simulink model "ps_model"  (R2023b)
settings: Solver=ode23tb  StartTime=0.0  StopTime=simlength  FixedStep=tc  MaxStep=tc
undefined symbols (not defined in the file): Amplitude_U, Amplitude_V, Amplitude_W, CFi, end_time_LVRT, fnom, fPWM_INV, i_nom, ki_i, ki_u, kp_i, kp_u, Ld2_trafo_out, magnitude, n10, number_of_cells, omega_grid_emulator_nom, Phase_shift, Q, q1Kalman, q2Kalman, q3Kalman, R_RLload, Rd2_trafo_out, rKalman, start_time_LVRT, t_ramp, tc, time_load_step, ts_afe, ts_inv, tsample, u_nom, ugrid_factor, V_phase_normalization_factor, Vdc_base, Vdc_nom, Vemu_ref_norm, vn_eta_pu, vn_xi_pu, vp_xi_pu
libraries: fl_lib x120, nesl_utility x67, cstblocks x8, ee_lib x7, single_phase_transformer_lib x3, lithium_ion_cell_lib x1, simulink x1, threephase_inductor_lib x1
(part 1 of 4)
settings Model: SimulationMode=accelerator  Creator=dbagn  LastModifiedBy=dbagn
settings SolverCC: NumberNewtonIterations=3  ZeroCrossControl=DisableAll  AlgebraicLoopSolver=TrustRegion  SolverResetMethod=Robust
settings DataIOCC: SaveOutput=off  SignalLogging=off  DSMLogging=off  SaveTime=off  ReturnWorkspaceOutputs=off
settings OptimizationCC: ReuseModelBlockBuffer=off
settings DebuggingCC: UnconnectedInputMsg=warning  UnconnectedOutputMsg=warning  UnconnectedLineMsg=warning
settings ModelReferenceCC: EnableRefExpFcnMdlSchedulingChecks=on
settings SFSimCC: SimUserIncludeDirs=include  SimAnalyzeCustomCode=on
settings SFSimCC: SimCustomHeaderCode=|
  | #include "mavgflt.h"
  | #include "bemf_obsv.h"
  | #include "dqvector_pi.h"
  | #include "dqvector_pi_simulink.h"
  | #include "mavgflt_simulink.h"
  | #include "sv_pwm.h"
  | #include "bemf_obsv_simulink.h"
  | #include "bemf_obsv_redu.h"
  | #include "bemf_obsv_redu_simulink.h"
  | #include "bemf_obsv_load_est.h"
  | #include "bemf_obsv_load_est_simulink.h"
  | #include "bemf_obsv_load_est_redu.h"
  | #include "bemf_obsv_load_est_redu_simulink.h"
  | #include "sv_pwm_simulink.h"
  | #include "fb_state_machine.h"
  | #include "fb_state_machine_simulink.h"
settings SFSimCC: SimUserSources=|
  | dqvector_pi.c
  | dqvector_pi_simulink.c
  | mavgflt_simulink.c
  | mavgflt.c
  | bemf_obsv_simulink.c
  | bemf_obsv.c
  | bemf_obsv_redu_simulink.c
  | bemf_obsv_redu.c
  | bemf_obsv_load_est_simulink.c
  | bemf_obsv_load_est.c
  | bemf_obsv_load_est_redu_simulink.c
  | bemf_obsv_load_est_redu.c
  | sv_pwm.c
  | sv_pwm_simulink.c
  | fb_state_machine.c
  | fb_state_machine_simulink.c
settings RTWCC: DLArmComputeVersion=19.05

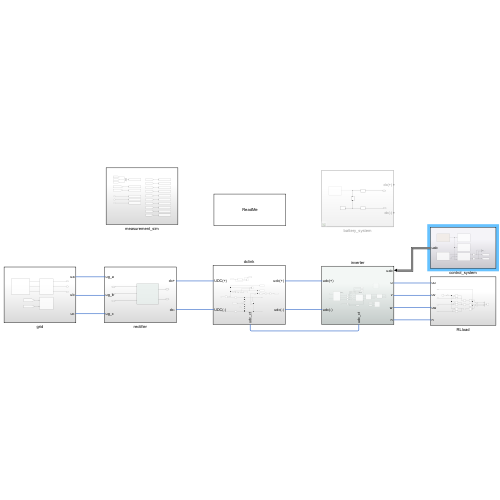
[thumbnail: Simulink's stored preview of the top-level diagram]
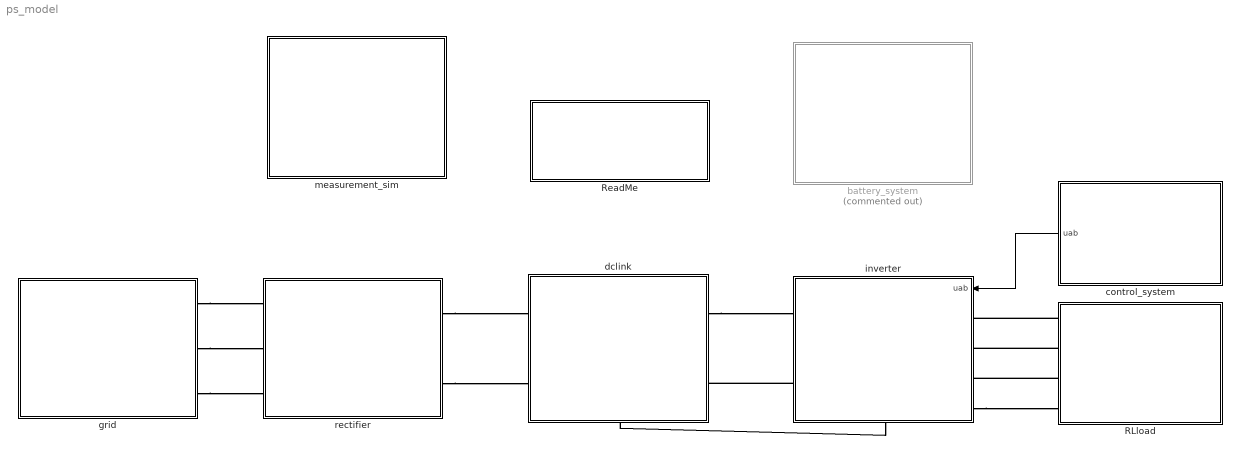
== system ps_model ==
  RLload : Subsystem
  ReadMe : Subsystem
      mask Display: disp('ReadMe')
  battery_system : Subsystem  Commented=on
  control_system : Subsystem
  dclink : Subsystem
      settings: PortSchema="{\"entries\":[{\"content\":{\"sides\":[{\"content\":{\"connectorIds\":[\"LConn1\",\"LConn2\"]},\"type\":\"ConnectorPlacement.EquallySpacedRectSide\",\"uuid\":\"065d3cf8-4b88-4bd8-afed-5c791b4c8227\"},{\"content\":{\"connectorIds\":[\"RConn1\",\"RConn2\"],\"side\":\"RIGHT\"},\"type\":\"ConnectorPlacement.EquallySpacedRectSide\",\"uuid\":\"93da4eee-d833-4749-b194-724bf2a8184c\"},{\"content\":{\"side\":\"TOP\"},\"type\":\"ConnectorPlacement.EquallySpacedRectSide\",\"uuid\":\"7e72ab0b-6fa9-40de-a645-1ec9cfd9e31f\"},{\"content\":{\"connectorIds\":[\"RConn3\"],\"side\":\"BOTTOM\"},\"type\":\"ConnectorPlacement.EquallySpacedRectSide\",\"uuid\":\"310375c4-299b-412a-a0fa-962bdc2b4f11\"}]},\"type\":\"ConnectorPlacement.EquallySpacedConnector\",\"uuid\":\"547429aa-4b93-405e-bc45-7aab171afd7d\"}],\"packageUris\":[\"http://schema.mathworks.com/mf0/Connector/R2020b\"],\"version\":\"1.0\"}"
  grid : Subsystem
  inverter : Subsystem
      settings: PortSchema="{\"entries\":[{\"content\":{\"sides\":[{\"content\":{\"connectorIds\":[\"In1\",\"LConn1\",\"LConn2\",\"LConn3\",\"LConn4\"]},\"type\":\"ConnectorPlacement.EquallySpacedRectSide\",\"uuid\":\"f55c1ca8-6919-4d30-91be-29ab6e5a5b93\"},{\"content\":{\"connectorIds\":[\"RConn1\",\"RConn2\"],\"side\":\"RIGHT\"},\"type\":\"ConnectorPlacement.EquallySpacedRectSide\",\"uuid\":\"500f40ac-770d-4aaa-b814-72c952c48909\"},{\"content\":{\"side\":\"TOP\"},\"type\":\"ConnectorPlacement.EquallySpacedRectSide\",\"uuid\":\"36360c7a-d142-42b5-a71d-dca271faa73f\"},{\"content\":{\"connectorIds\":[\"RConn3\"],\"side\":\"BOTTOM\"},\"type\":\"ConnectorPlacement.EquallySpacedRectSide\",\"uuid\":\"19fec778-0473-49a4-aa84-7932c0a6b289\"}]},\"type\":\"ConnectorPlacement.EquallySpacedConnector\",\"uuid\":\"7d88957d-a3a4-4eee-9ba8-53fe19feea5c\"}],\"packageUris\":[\"http://schema.mathworks.com/mf0/Connector/R2020b\"],\"version\":\"1.0\"}"
  measurement_sim : Subsystem
  rectifier : Subsystem
  wires:
  control_system/1(uab) -> inverter/1(uab)
  connections:
  rectifier/RConn1 -- dclink/LConn1
  rectifier/RConn2 -- dclink/LConn2
  inverter/RConn2 -- dclink/RConn2
  dclink/RConn1 -- inverter/RConn1
  RLload/LConn3 -- inverter/LConn3
  RLload/LConn2 -- inverter/LConn2
  RLload/LConn1 -- inverter/LConn1
  grid/RConn1 -- rectifier/LConn1
  grid/RConn2 -- rectifier/LConn2
  grid/RConn3 -- rectifier/LConn3
  inverter/RConn3 -- dclink/RConn3
  inverter/LConn4 -- RLload/LConn4

== system ps_model/RLload ==
  Bus Creator1 : BusCreator  Inputs=3
  Current Sensor : fl_lib/Electrical/Electrical Sensors/Current Sensor
  Current Sensor1 : fl_lib/Electrical/Electrical Sensors/Current Sensor
  Current Sensor2 : fl_lib/Electrical/Electrical Sensors/Current Sensor
  Inductor : ee_lib/Passive/Inductor  l=L_RLload H  enable_L_tol=0  L_tol=20  tol_distribution=1  nSigma=4  r=0 Ohm  g=1e-9 1/Ohm  enable_operating_limits=0  operating_limit_action=2  max_working_current=1 A  power_rating=1 W  enable_faults=ee.enum.enable.no  fault_action=simscape.enum.assert.action.none  lambdaPercent=50  k_faulted=0.9999  turnsShort=0  openCct=0  groundShort=0  groundShortG=0 1/Ohm  tau_fault=1e-3 s  fault_trigger=ee.enum.faults.faultTrigger.temporal  t_fault=1 s  max_permissible_voltage=100 V  n_fail_on_voltage=1  max_permissible_current=1 A  t_fail_on_current=1 s  i_L_specify=off  i_L_priority=High  i_L=0 A  i_L_nominal_specify=off  i_L_nominal_unit=A  i_L_nominal_value=1
  Inductor1 : ee_lib/Passive/Inductor  l=L_RLload H  enable_L_tol=0  L_tol=20  tol_distribution=1  nSigma=4  r=0 Ohm  g=1e-9 1/Ohm  enable_operating_limits=0  operating_limit_action=2  max_working_current=1 A  power_rating=1 W  enable_faults=ee.enum.enable.no  fault_action=simscape.enum.assert.action.none  lambdaPercent=50  k_faulted=0.9999  turnsShort=0  openCct=0  groundShort=0  groundShortG=0 1/Ohm  tau_fault=1e-3 s  fault_trigger=ee.enum.faults.faultTrigger.temporal  t_fault=1 s  max_permissible_voltage=100 V  n_fail_on_voltage=1  max_permissible_current=1 A  t_fail_on_current=1 s  i_L_specify=off  i_L_priority=High  i_L=0 A  i_L_nominal_specify=off  i_L_nominal_unit=A  i_L_nominal_value=1
  Inductor2 : ee_lib/Passive/Inductor  l=L_RLload H  enable_L_tol=0  L_tol=20  tol_distribution=1  nSigma=4  r=0 Ohm  g=1e-9 1/Ohm  enable_operating_limits=0  operating_limit_action=2  max_working_current=1 A  power_rating=1 W  enable_faults=ee.enum.enable.no  fault_action=simscape.enum.assert.action.none  lambdaPercent=50  k_faulted=0.9999  turnsShort=0  openCct=0  groundShort=0  groundShortG=0 1/Ohm  tau_fault=1e-3 s  fault_trigger=ee.enum.faults.faultTrigger.temporal  t_fault=1 s  max_permissible_voltage=100 V  n_fail_on_voltage=1  max_permissible_current=1 A  t_fail_on_current=1 s  i_L_specify=off  i_L_priority=High  i_L=0 A  i_L_nominal_specify=off  i_L_nominal_unit=A  i_L_nominal_value=1
  PS-Simulink Converter1 : nesl_utility/PS-Simulink Converter  PhysicalDomain=network_engine_domain  SubClassName=ps_output  LeftPortType=input  RightPortType=output  PseudoPeriodic=off  Frequencies=[]  VectorFormat=1-D array  Unit=A  AffineConversion=off
  PS-Simulink Converter2 : nesl_utility/PS-Simulink Converter  PhysicalDomain=network_engine_domain  SubClassName=ps_output  LeftPortType=input  RightPortType=output  PseudoPeriodic=off  Frequencies=[]  VectorFormat=1-D array  Unit=A  AffineConversion=off
  PS-Simulink Converter3 : nesl_utility/PS-Simulink Converter  PhysicalDomain=network_engine_domain  SubClassName=ps_output  LeftPortType=input  RightPortType=output  PseudoPeriodic=off  Frequencies=[]  VectorFormat=1-D array  Unit=A  AffineConversion=off
  Resistor : fl_lib/Electrical/Electrical Elements/Resistor  R=R_RLload Ohm  i_specify=off  i_priority=None  i=0 A  i_nominal_specify=off  i_nominal_unit=A  i_nominal_value=1  v_specify=off  v_priority=None  v=0 V  v_nominal_specify=off  v_nominal_unit=V  v_nominal_value=1
  Resistor1 : fl_lib/Electrical/Electrical Elements/Resistor  R=R_RLload Ohm  i_specify=off  i_priority=None  i=0 A  i_nominal_specify=off  i_nominal_unit=A  i_nominal_value=1  v_specify=off  v_priority=None  v=0 V  v_nominal_specify=off  v_nominal_unit=V  v_nominal_value=1
  Resistor2 : fl_lib/Electrical/Electrical Elements/Resistor  R=R_RLload Ohm  i_specify=off  i_priority=None  i=0 A  i_nominal_specify=off  i_nominal_unit=A  i_nominal_value=1  v_specify=off  v_priority=None  v=0 V  v_nominal_specify=off  v_nominal_unit=V  v_nominal_value=1
  Simulink-PS Converter : nesl_utility/Simulink-PS Converter  PhysicalDomain=network_engine_domain  SubClassName=ps_input  LeftPortType=input  RightPortType=output  PseudoPeriodic=off  Frequencies=[]  NoiseDistribution=none  NoiseParameters=[]  Unit=1  AffineConversion=off  FilteringAndDerivatives=provide  SimscapeFilterOrder=1  InputFilterTimeConstant=0.001  UdotUserProvided=0
  Step : Step  Time=time_load_step  SampleTime=0
  Switch : fl_lib/Electrical/Electrical Elements/Switch  R_closed=0.8 Ohm  G_open=1e-8 1/Ohm  Threshold=0.5  i_specify=off  i_priority=None  i=0 A  i_nominal_specify=off  i_nominal_unit=A  i_nominal_value=1  v_specify=off  v_priority=None  v=0 V  v_nominal_specify=off  v_nominal_unit=V  v_nominal_value=1
  Switch1 : fl_lib/Electrical/Electrical Elements/Switch  R_closed=0.8 Ohm  G_open=1e-8 1/Ohm  Threshold=0.5  i_specify=off  i_priority=None  i=0 A  i_nominal_specify=off  i_nominal_unit=A  i_nominal_value=1  v_specify=off  v_priority=None  v=0 V  v_nominal_specify=off  v_nominal_unit=V  v_nominal_value=1
  Switch2 : fl_lib/Electrical/Electrical Elements/Switch  R_closed=0.8 Ohm  G_open=1e-8 1/Ohm  Threshold=0.5  i_specify=off  i_priority=None  i=0 A  i_nominal_specify=off  i_nominal_unit=A  i_nominal_value=1  v_specify=off  v_priority=None  v=0 V  v_nominal_specify=off  v_nominal_unit=V  v_nominal_value=1
  iuvw_load : Scope
  uu : PMIOPort  Side=Left
  uv : PMIOPort  Port=2  Side=Left
  uw : PMIOPort  Port=3  Side=Left
  n : PMIOPort  Port=4  Side=Left
  wires:
  PS-Simulink Converter1/1 -> Bus Creator1/1  "iu_load_sim"
  Bus Creator1/1 -> iuvw_load/1
  PS-Simulink Converter3/1 -> Bus Creator1/3  "iw_load_sim"
  PS-Simulink Converter2/1 -> Bus Creator1/2  "iv_load_sim"
  Step/1 -> Simulink-PS Converter/1
  connections:
  uv/RConn1 -- Switch1/RConn2 -- Resistor1/LConn1
  Resistor/LConn1 -- uu/RConn1 -- Switch/RConn2
  uw/RConn1 -- Switch2/RConn2 -- Resistor2/LConn1
  Resistor1/RConn1 -- Switch1/LConn1 -- Inductor1/LConn1
  Switch/LConn1 -- Resistor/RConn1 -- Inductor/LConn1
  Inductor2/LConn1 -- Switch2/LConn1 -- Resistor2/RConn1
  PS-Simulink Converter3/LConn1 -- Current Sensor2/RConn1
  Current Sensor1/RConn1 -- PS-Simulink Converter2/LConn1
  Current Sensor/RConn2 -- Current Sensor2/RConn2 -- Current Sensor1/RConn2 -- n/RConn1
  Current Sensor/RConn1 -- PS-Simulink Converter1/LConn1
  Current Sensor/LConn1 -- Inductor/RConn1
  Inductor2/RConn1 -- Current Sensor2/LConn1
  Inductor1/RConn1 -- Current Sensor1/LConn1
  Switch/RConn1 -- Simulink-PS Converter/RConn1 -- Switch2/RConn1 -- Switch1/RConn1

== system ps_model/ReadMe ==

== system ps_model/battery_system ==
  DC Voltage Source : fl_lib/Electrical/Electrical Sources/DC Voltage Source  v0=Vdc_ref V
  Inductor : fl_lib/Electrical/Electrical Elements/Inductor  l=100e-6 H  r=0.025 Ohm  g=1e-9 1/Ohm  i_specify=off  i_priority=None  i=0 A  i_nominal_specify=off  i_nominal_unit=A  i_nominal_value=1  v_specify=off  v_priority=None  v=0 V  v_nominal_specify=off  v_nominal_unit=V  v_nominal_value=1  i_L_specify=off  i_L_priority=High  i_L=0 A  i_L_nominal_specify=off  i_L_nominal_unit=A  i_L_nominal_value=1
  Inductor1 : fl_lib/Electrical/Electrical Elements/Inductor  l=100e-6 H  r=0.025 Ohm  g=1e-9 1/Ohm  i_specify=off  i_priority=None  i=0 A  i_nominal_specify=off  i_nominal_unit=A  i_nominal_value=1  v_specify=off  v_priority=None  v=0 V  v_nominal_specify=off  v_nominal_unit=V  v_nominal_value=1  i_L_specify=off  i_L_priority=High  i_L=0 A  i_L_nominal_specify=off  i_L_nominal_unit=A  i_L_nominal_value=1
  Solver Configuration : nesl_utility/Solver Configuration  PhysicalDomain=network_engine_domain  SubClassName=solver  LeftPortType=input  RightPortType=generic  Tones=[]  Harmonics=[]  SimulateNoise=off  Profile=off  UseLocalSampling=off  EnableSwitchedLinearOptims=on  FrequencyDomain=off  UseCCode=off  RelTol=0.001  AbsTol=0.001  MinStep=1e-09  ToWorkspace=off  RevertToSquareIcSolve=off  NumHomotopyIterations=100  PhasorMode=off  PhasorModeNumHarmonics=1  ConsistencySolver=NEWTON_FTOL  IndexReductionMethod=DerivativeReplacement  DoDC=off  ResidualTolerance=1e-09  ConsistencyTolSource=GLOBAL  ConsistencyAbsTol=0.001  ConsistencyRelTol=0.001  ConsistencyTolFactor=0.001  UseLocalSolver=on  LocalSolverChoice=NE_BACKWARD_EULER_ADVANCER  ResolveIndetEquations=on  FunctionEvalNumThread=1  LocalSolverSampleTime=tc  DoFixedCost=on  MaxNonlinIter=5  MaxModeIter=2  ComputeImpulses=off  ImpulseIterations=2  LinearAlgebra=auto  LinearAlgebraNumThread=0  EquationFormulation=NE_TIME_EF  DelaysMemoryBudget=1024  AutomaticFiltering=on  FilteringTimeConstant=0.001  PartitionStorageMethod=AS_NEEDED  PartitionMemoryBudget=1024  PartitionMethod=ROBUST  MultibodyUseLocalSolver=off  MultibodyLocalSolverChoice=ODE1  MultibodyLocalSolverSampleTime=0.001
  battery_system : Subsystem  Commented=on
  dc(+) : PMIOPort  Side=Right
  dc(-) : PMIOPort  Port=2  Side=Right
  connections:
  Solver Configuration/RConn1 -- Inductor1/LConn1 -- DC Voltage Source/RConn1
  DC Voltage Source/LConn1 -- Inductor/LConn1 -- battery_system/RConn1
  Inductor/RConn1 -- dc(+)/RConn1
  Inductor1/RConn1 -- dc(-)/RConn1

== system ps_model/control_system ==
  Bus Creator1 : BusCreator  Inputs=2
  Unit Delay1 : UnitDelay  SampleTime=ts_inv  HasFrameUpgradeWarning=on
  Unit Delay2 : UnitDelay  SampleTime=ts_inv  HasFrameUpgradeWarning=on
  current_measure : Subsystem
  dq2alphabeta : MATLAB Function  TreatAsAtomicUnit=on  SystemSampleTime=ts_inv
  phase_gen : Subsystem
  scalar_voltage_control : Subsystem
  voltage_measure : Subsystem
  uab : Outport  VectorParamsAs1DForOutWhenUnconnected=off
  tag scope: u_alpha_ctrl_out=global, u_beta_ctrl_out=global
  wires:
  Unit Delay1/1 -> [u_alpha_ctrl_out], Bus Creator1/1  "ua"
  phase_gen/1(electrical_phase) -> current_measure/1(phase), voltage_measure/1(phase), dq2alphabeta/3(phase)
  Unit Delay2/1 -> [u_beta_ctrl_out], Bus Creator1/2  "ub"
  dq2alphabeta/1(alpha) -> Unit Delay1/1  "ua"
  Bus Creator1/1 -> uab/1
  dq2alphabeta/2(beta) -> Unit Delay2/1  "ub"
  scalar_voltage_control/1(d) -> dq2alphabeta/1(d)
  scalar_voltage_control/2(q) -> dq2alphabeta/2(q)

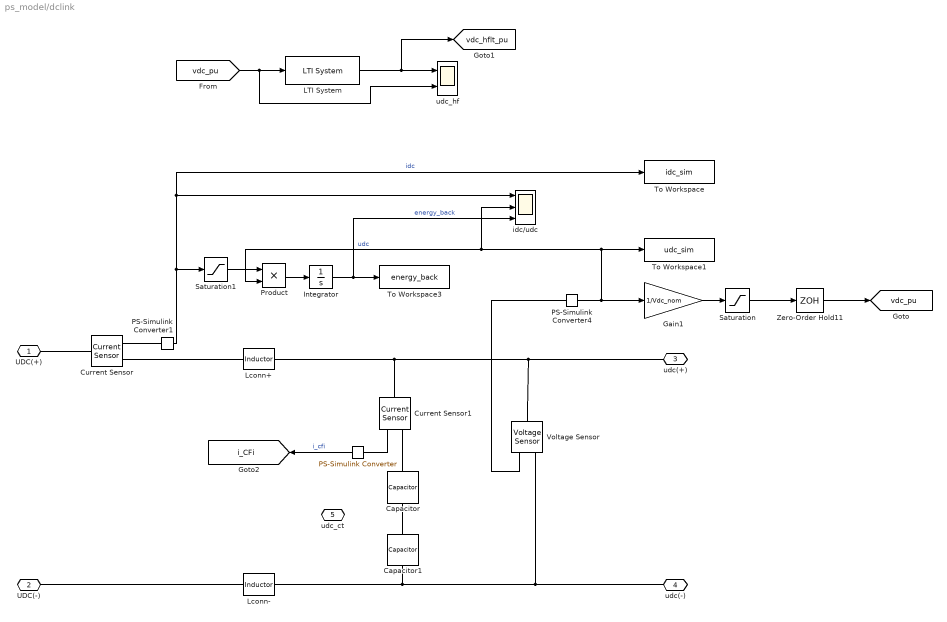
== system ps_model/dclink ==
  " " : nesl_utility/PS-Simulink Converter  PhysicalDomain=network_engine_domain  SubClassName=ps_output  LeftPortType=input  RightPortType=output  PseudoPeriodic=off  Frequencies=[]  VectorFormat=1-D array  Unit=A  AffineConversion=off
  Capacitor : fl_lib/Electrical/Electrical Elements/Capacitor  c=2*CFi F  r=1e-3 Ohm  g=0 1/Ohm  i_specify=off  i_priority=None  i=0 A  i_nominal_specify=off  i_nominal_unit=A  i_nominal_value=1  v_specify=off  v_priority=None  v=0 V  v_nominal_specify=off  v_nominal_unit=V  v_nominal_value=1  vc_specify=off  vc_priority=High  vc=0 V  vc_nominal_specify=off  vc_nominal_unit=V  vc_nominal_value=1
  Capacitor1 : fl_lib/Electrical/Electrical Elements/Capacitor  c=2*CFi F  r=1e-3 Ohm  g=0 1/Ohm  i_specify=off  i_priority=None  i=0 A  i_nominal_specify=off  i_nominal_unit=A  i_nominal_value=1  v_specify=off  v_priority=None  v=0 V  v_nominal_specify=off  v_nominal_unit=V  v_nominal_value=1  vc_specify=off  vc_priority=High  vc=0 V  vc_nominal_specify=off  vc_nominal_unit=V  vc_nominal_value=1
  Current Sensor : fl_lib/Electrical/Electrical Sensors/Current Sensor
  Current Sensor1 : fl_lib/Electrical/Electrical Sensors/Current Sensor
  Gain1 : Gain  Gain=1/Vdc_nom
  Integrator : Integrator
  LTI System : cstblocks/LTI System  sys=hpf2q_d  IC=[]  PadeOrder=0
  Lconn+ : fl_lib/Electrical/Electrical Elements/Inductor  l=0.5e-6 H  r=5e-3 Ohm  g=1e-9 1/Ohm  i_specify=on  i_priority=High  i=0 A  i_nominal_specify=off  i_nominal_unit=A  i_nominal_value=1  v_specify=off  v_priority=None  v=0 V  v_nominal_specify=off  v_nominal_unit=V  v_nominal_value=1  i_L_specify=off  i_L_priority=High  i_L=0 A  i_L_nominal_specify=off  i_L_nominal_unit=A  i_L_nominal_value=1
  Lconn- : fl_lib/Electrical/Electrical Elements/Inductor  l=0.5e-6 H  r=5e-3 Ohm  g=1e-9 1/Ohm  i_specify=on  i_priority=High  i=0 A  i_nominal_specify=off  i_nominal_unit=A  i_nominal_value=1  v_specify=off  v_priority=None  v=0 V  v_nominal_specify=off  v_nominal_unit=V  v_nominal_value=1  i_L_specify=off  i_L_priority=High  i_L=0 A  i_L_nominal_specify=off  i_L_nominal_unit=A  i_L_nominal_value=1
  PS-Simulink Converter1 : nesl_utility/PS-Simulink Converter  PhysicalDomain=network_engine_domain  SubClassName=ps_output  LeftPortType=input  RightPortType=output  PseudoPeriodic=off  Frequencies=[]  VectorFormat=1-D array  Unit=A  AffineConversion=on
  PS-Simulink Converter4 : nesl_utility/PS-Simulink Converter  PhysicalDomain=network_engine_domain  SubClassName=ps_output  LeftPortType=input  RightPortType=output  PseudoPeriodic=off  Frequencies=[]  VectorFormat=1-D array  Unit=V  AffineConversion=on
  Product : Product
  Saturation : Saturate  UpperLimit=inf  LowerLimit=0.1
  Saturation1 : Saturate  UpperLimit=0  LowerLimit=-inf
  To Workspace : ToWorkspace  VariableName=idc_sim  SampleTime=tc
      settings: MaxDataPoints=Nc
  To Workspace1 : ToWorkspace  VariableName=udc_sim  SampleTime=tc
      settings: MaxDataPoints=Nc
  To Workspace3 : ToWorkspace  VariableName=energy_back  SampleTime=tc
      settings: MaxDataPoints=Nc
  Voltage Sensor : fl_lib/Electrical/Electrical Sensors/Voltage Sensor
  Zero-Order Hold11 : ZeroOrderHold  SampleTime=ts_inv
  idc/udc : Scope  NumInputPorts=3
  udc_hf : Scope  NumInputPorts=2
  UDC(+) : PMIOPort  Side=Left
  UDC(-) : PMIOPort  Port=2  Side=Left
  udc(+) : PMIOPort  Port=3  Side=Right
  udc(-) : PMIOPort  Port=4  Side=Right
  udc_ct : PMIOPort  Port=5  Side=Right
  tag scope: i_CFi=global, vdc_hflt_pu=global, vdc_pu=global
  wires:
  Saturation/1 -> Zero-Order Hold11/1
  PS-Simulink Converter4/1 -> idc/udc/2, Product/2, To Workspace1/1, Gain1/1  "udc"
  Gain1/1 -> Saturation/1
  PS-Simulink Converter1/1 -> Saturation1/1, To Workspace/1, idc/udc/1  "idc"
  Saturation1/1 -> Product/1
  Product/1 -> Integrator/1
  Integrator/1 -> idc/udc/3, To Workspace3/1  "energy_back"
  LTI System/1 -> [vdc_hflt_pu], udc_hf/1
  [vdc_pu] -> udc_hf/2, LTI System/1
  Zero-Order Hold11/1 -> [vdc_pu]
  " "/1 -> [i_CFi]  "i_cfi"
  connections:
  PS-Simulink Converter4/LConn1 -- Voltage Sensor/RConn1
  PS-Simulink Converter1/LConn1 -- Current Sensor/RConn1
  Current Sensor/RConn2 -- Lconn+/LConn1
  Current Sensor/LConn1 -- UDC(+)/RConn1
  Lconn-/RConn1 -- UDC(-)/RConn1
  Lconn+/RConn1 -- Current Sensor1/LConn1 -- Voltage Sensor/LConn1 -- udc(+)/RConn1
  Voltage Sensor/RConn2 -- udc(-)/RConn1 -- Capacitor1/RConn1 -- Lconn-/LConn1
  Capacitor1/LConn1 -- Capacitor/RConn1
  Current Sensor1/RConn1 -- " "/LConn1
  Current Sensor1/RConn2 -- Capacitor/LConn1

== system ps_model/grid ==
  grid_emulator : Subsystem
  instantaneus_power : Subsystem
  threephase_vi_measures : Subsystem
  ua : PMIOPort  Side=Right
  ub : PMIOPort  Port=2  Side=Right
  uc : PMIOPort  Port=3  Side=Right
  wires:
  [vgrid_abc] -> instantaneus_power/1(Vline)
  [igrid_abc] -> instantaneus_power/2(Iline)
  connections:
  threephase_vi_measures/LConn3 -- grid_emulator/RConn3
  threephase_vi_measures/LConn1 -- grid_emulator/RConn1
  threephase_vi_measures/RConn2 -- ub/RConn1
  threephase_vi_measures/LConn2 -- grid_emulator/RConn2
  threephase_vi_measures/RConn1 -- ua/RConn1
  threephase_vi_measures/RConn3 -- uc/RConn1

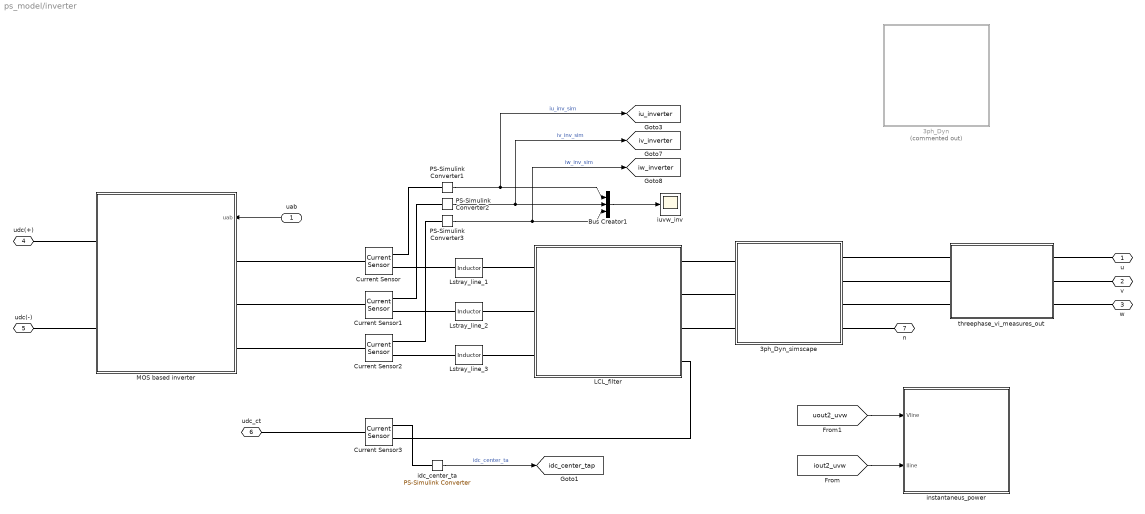
== system ps_model/inverter ==
  uab : Inport
  3ph_Dyn : Subsystem  Commented=on
  3ph_Dyn_simscape : Subsystem
  Bus Creator1 : BusCreator  Inputs=3
  Current Sensor{,1..3} (4 alike) : fl_lib/Electrical/Electrical Sensors/Current Sensor
  LCL_filter : Subsystem
  Lstray_line_1 : ee_lib/Passive/Inductor  l=5e-6 H  enable_L_tol=ee.enum.toleranceApplication.none  L_tol=20  tol_distribution=ee.enum.toleranceDistribution.uniform  nSigma=4  r=0 Ohm  g=1e-9 1/Ohm  enable_operating_limits=ee.enum.enable.no  operating_limit_action=ee.enum.passive.reportOpLim.warn  max_working_current=1 A  power_rating=1 W  enable_faults=ee.enum.enable.no  fault_action=simscape.enum.assert.action.none  lambdaPercent=50  k_faulted=0.9999  turnsShort=ee.enum.passive.inductor.turnsShortOption.no  openCct=ee.enum.enable.no  groundShort=ee.enum.passive.inductor.groundShortOption.no  groundShortG=0 1/Ohm  tau_fault=1e-3 s  fault_trigger=ee.enum.faults.faultTrigger.temporal  t_fault=1 s  max_permissible_voltage=100 V  n_fail_on_voltage=1  max_permissible_current=1 A  t_fail_on_current=1 s  i_L_specify=on  i_L_priority=High  i_L=0 A  i_L_nominal_specify=off  i_L_nominal_unit=A  i_L_nominal_value=1
  Lstray_line_2 : ee_lib/Passive/Inductor  l=5e-6 H  enable_L_tol=ee.enum.toleranceApplication.none  L_tol=20  tol_distribution=ee.enum.toleranceDistribution.uniform  nSigma=4  r=0 Ohm  g=1e-9 1/Ohm  enable_operating_limits=ee.enum.enable.no  operating_limit_action=ee.enum.passive.reportOpLim.warn  max_working_current=1 A  power_rating=1 W  enable_faults=ee.enum.enable.no  fault_action=simscape.enum.assert.action.none  lambdaPercent=50  k_faulted=0.9999  turnsShort=ee.enum.passive.inductor.turnsShortOption.no  openCct=ee.enum.enable.no  groundShort=ee.enum.passive.inductor.groundShortOption.no  groundShortG=0 1/Ohm  tau_fault=1e-3 s  fault_trigger=ee.enum.faults.faultTrigger.temporal  t_fault=1 s  max_permissible_voltage=100 V  n_fail_on_voltage=1  max_permissible_current=1 A  t_fail_on_current=1 s  i_L_specify=on  i_L_priority=High  i_L=0 A  i_L_nominal_specify=off  i_L_nominal_unit=A  i_L_nominal_value=1
  Lstray_line_3 : ee_lib/Passive/Inductor  l=5e-6 H  enable_L_tol=ee.enum.toleranceApplication.none  L_tol=20  tol_distribution=ee.enum.toleranceDistribution.uniform  nSigma=4  r=0 Ohm  g=1e-9 1/Ohm  enable_operating_limits=ee.enum.enable.no  operating_limit_action=ee.enum.passive.reportOpLim.warn  max_working_current=1 A  power_rating=1 W  enable_faults=ee.enum.enable.no  fault_action=simscape.enum.assert.action.none  lambdaPercent=50  k_faulted=0.9999  turnsShort=ee.enum.passive.inductor.turnsShortOption.no  openCct=ee.enum.enable.no  groundShort=ee.enum.passive.inductor.groundShortOption.no  groundShortG=0 1/Ohm  tau_fault=1e-3 s  fault_trigger=ee.enum.faults.faultTrigger.temporal  t_fault=1 s  max_permissible_voltage=100 V  n_fail_on_voltage=1  max_permissible_current=1 A  t_fail_on_current=1 s  i_L_specify=on  i_L_priority=High  i_L=0 A  i_L_nominal_specify=off  i_L_nominal_unit=A  i_L_nominal_value=1
  MOS based inverter : Subsystem
  PS-Simulink Converter1 : nesl_utility/PS-Simulink Converter  PhysicalDomain=network_engine_domain  SubClassName=ps_output  LeftPortType=input  RightPortType=output  PseudoPeriodic=off  Frequencies=[]  VectorFormat=1-D array  Unit=A  AffineConversion=off
  PS-Simulink Converter2 : nesl_utility/PS-Simulink Converter  PhysicalDomain=network_engine_domain  SubClassName=ps_output  LeftPortType=input  RightPortType=output  PseudoPeriodic=off  Frequencies=[]  VectorFormat=1-D array  Unit=A  AffineConversion=off
  PS-Simulink Converter3 : nesl_utility/PS-Simulink Converter  PhysicalDomain=network_engine_domain  SubClassName=ps_output  LeftPortType=input  RightPortType=output  PseudoPeriodic=off  Frequencies=[]  VectorFormat=1-D array  Unit=A  AffineConversion=off
  idc_center_ta : nesl_utility/PS-Simulink Converter  PhysicalDomain=network_engine_domain  SubClassName=ps_output  LeftPortType=input  RightPortType=output  PseudoPeriodic=off  Frequencies=[]  VectorFormat=1-D array  Unit=A  AffineConversion=off
  instantaneus_power : Subsystem
  iuvw_inv : Scope
  threephase_vi_measures_out : Subsystem
  u : PMIOPort  Side=Left
  v : PMIOPort  Port=2  Side=Left
  w : PMIOPort  Port=3  Side=Left
  udc(+) : PMIOPort  Port=4  Side=Right
  udc(-) : PMIOPort  Port=5  Side=Right
  udc_ct : PMIOPort  Port=6  Side=Right
  n : PMIOPort  Port=7  Side=Left
  tag scope: idc_center_tap=global, iu_inverter=global, iv_inverter=global, iw_inverter=global
  wires:
  Bus Creator1/1 -> iuvw_inv/1
  PS-Simulink Converter3/1 -> Bus Creator1/3, [iw_inverter]  "iw_inv_sim"
  PS-Simulink Converter1/1 -> [iu_inverter], Bus Creator1/1  "iu_inv_sim"
  PS-Simulink Converter2/1 -> [iv_inverter], Bus Creator1/2  "iv_inv_sim"
  uab/1 -> MOS based inverter/1(uab)
  idc_center_ta/1 -> [idc_center_tap]  "idc_center_ta"
  [iout2_uvw] -> instantaneus_power/2(Iline)
  [uout2_uvw] -> instantaneus_power/1(Vline)
  connections:
  Current Sensor1/LConn1 -- MOS based inverter/LConn2
  Current Sensor/LConn1 -- MOS based inverter/LConn1
  Current Sensor2/LConn1 -- MOS based inverter/LConn3
  udc(+)/RConn1 -- MOS based inverter/RConn1
  udc(-)/RConn1 -- MOS based inverter/RConn2
  PS-Simulink Converter3/LConn1 -- Current Sensor2/RConn1
  Current Sensor1/RConn1 -- PS-Simulink Converter2/LConn1
  Current Sensor1/RConn2 -- Lstray_line_2/LConn1
  Current Sensor/RConn1 -- PS-Simulink Converter1/LConn1
  Current Sensor/RConn2 -- Lstray_line_1/LConn1
  Current Sensor2/RConn2 -- Lstray_line_3/LConn1
  LCL_filter/LConn1 -- Lstray_line_1/RConn1
  LCL_filter/LConn2 -- Lstray_line_2/RConn1
  LCL_filter/LConn3 -- Lstray_line_3/RConn1
  threephase_vi_measures_out/RConn1 -- u/RConn1
  threephase_vi_measures_out/RConn2 -- v/RConn1
  threephase_vi_measures_out/RConn3 -- w/RConn1
  Current Sensor3/RConn2 -- LCL_filter/RConn4
  Current Sensor3/RConn1 -- idc_center_ta/LConn1
  udc_ct/RConn1 -- Current Sensor3/LConn1
  3ph_Dyn_simscape/RConn1 -- threephase_vi_measures_out/LConn1
  3ph_Dyn_simscape/LConn1 -- LCL_filter/RConn1
  3ph_Dyn_simscape/RConn2 -- threephase_vi_measures_out/LConn2
  3ph_Dyn_simscape/LConn2 -- LCL_filter/RConn2
  3ph_Dyn_simscape/RConn3 -- threephase_vi_measures_out/LConn3
  3ph_Dyn_simscape/LConn3 -- LCL_filter/RConn3
  3ph_Dyn_simscape/RConn4 -- n/RConn1

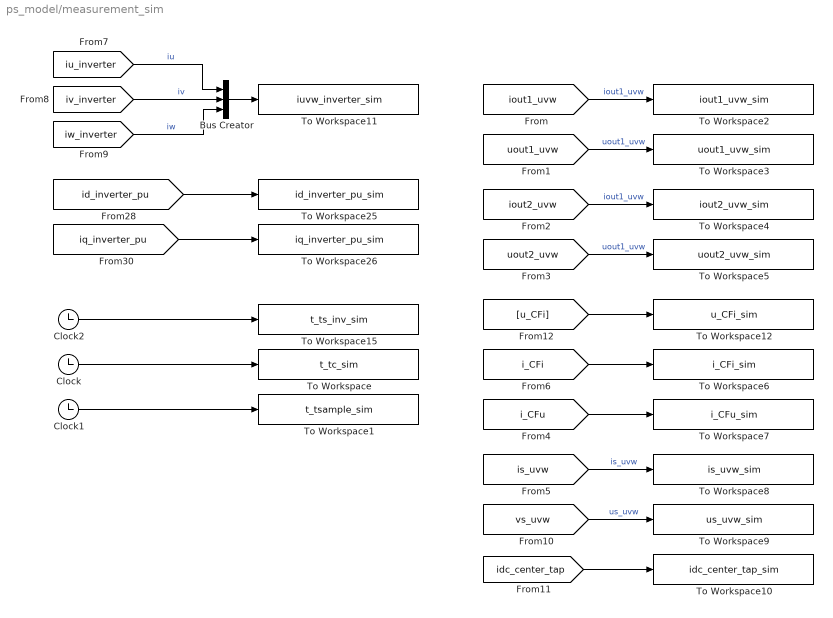
== system ps_model/measurement_sim ==
  Bus Creator : BusCreator  Inputs=3
  Clock : Clock
  Clock1 : Clock
  Clock2 : Clock
  To Workspace : ToWorkspace  VariableName=t_tc_sim  SampleTime=tc
      settings: MaxDataPoints=Nc
  To Workspace1 : ToWorkspace  VariableName=t_tsample_sim  SampleTime=tsample
      settings: MaxDataPoints=Nsample
  To Workspace10 : ToWorkspace  VariableName=idc_center_tap_sim  SampleTime=tc
      settings: MaxDataPoints=Nc
  To Workspace11 : ToWorkspace  VariableName=iuvw_inverter_sim  SampleTime=tc
      settings: MaxDataPoints=Nc
  To Workspace12 : ToWorkspace  VariableName=u_CFi_sim  SampleTime=tc
      settings: MaxDataPoints=Nc
  To Workspace15 : ToWorkspace  VariableName=t_ts_inv_sim  SampleTime=ts_inv
      settings: MaxDataPoints=Ns_inv
  To Workspace2 : ToWorkspace  VariableName=iout1_uvw_sim  SampleTime=tc
      settings: MaxDataPoints=Nc
  To Workspace25 : ToWorkspace  VariableName=id_inverter_pu_sim  SampleTime=tc
      settings: MaxDataPoints=Nc
  To Workspace26 : ToWorkspace  VariableName=iq_inverter_pu_sim  SampleTime=tc
      settings: MaxDataPoints=Nc
  To Workspace3 : ToWorkspace  VariableName=uout1_uvw_sim  SampleTime=tc
      settings: MaxDataPoints=Nc
  To Workspace4 : ToWorkspace  VariableName=iout2_uvw_sim  SampleTime=tc
      settings: MaxDataPoints=Nc
  To Workspace5 : ToWorkspace  VariableName=uout2_uvw_sim  SampleTime=tc
      settings: MaxDataPoints=Nc
  To Workspace6 : ToWorkspace  VariableName=i_CFi_sim  SampleTime=tc
      settings: MaxDataPoints=Nc
  To Workspace7 : ToWorkspace  VariableName=i_CFu_sim  SampleTime=tc
      settings: MaxDataPoints=Nc
  To Workspace8 : ToWorkspace  VariableName=is_uvw_sim  SampleTime=tc
      settings: MaxDataPoints=Nc
  To Workspace9 : ToWorkspace  VariableName=us_uvw_sim  SampleTime=tc
      settings: MaxDataPoints=Nc
  wires:
  Clock1/1 -> To Workspace1/1
  Clock/1 -> To Workspace/1
  [iv_inverter] -> Bus Creator/2  "iv"
  [iw_inverter] -> Bus Creator/3  "iw"
  [iu_inverter] -> Bus Creator/1  "iu"
  Bus Creator/1 -> To Workspace11/1
  Clock2/1 -> To Workspace15/1
  [id_inverter_pu] -> To Workspace25/1
  [iq_inverter_pu] -> To Workspace26/1
  [iout1_uvw] -> To Workspace2/1  "iout1_uvw"
  [uout1_uvw] -> To Workspace3/1  "uout1_uvw"
  [uout2_uvw] -> To Workspace5/1  "uout1_uvw"
  [iout2_uvw] -> To Workspace4/1  "iout1_uvw"
  [i_CFi] -> To Workspace6/1
  [i_CFu] -> To Workspace7/1
  [is_uvw] -> To Workspace8/1  "is_uvw"
  [vs_uvw] -> To Workspace9/1  "us_uvw"
  [idc_center_tap] -> To Workspace10/1
  [u_CFi] -> To Workspace12/1

== system ps_model/rectifier ==
  rectifier : Subsystem
  ug_a : PMIOPort  Side=Left
  dc+ : PMIOPort  Port=2  Side=Right
  ug_b : PMIOPort  Port=3  Side=Left
  dc- : PMIOPort  Port=4  Side=Right
  ug_c : PMIOPort  Port=5  Side=Left
  connections:
  dc-/RConn1 -- rectifier/RConn2
  dc+/RConn1 -- rectifier/RConn1
  rectifier/LConn1 -- ug_a/RConn1
  rectifier/LConn2 -- ug_b/RConn1
  rectifier/LConn3 -- ug_c/RConn1

== system ps_model/battery_system/battery_system ==
  Electrical Reference1 : fl_lib/Electrical/Electrical Elements/Electrical Reference
  LithiumIonBattery : Subsystem
  Uout+ : PMIOPort  Side=Right
  connections:
  LithiumIonBattery/RConn2 -- Electrical Reference1/LConn1
  LithiumIonBattery/RConn1 -- Uout+/RConn1

== system ps_model/control_system/current_measure ==
  phase : Inport
  current_transformation : Subsystem
  sample_hold_normalization : Subsystem
  wires:
  sample_hold_normalization/3(iw_pu) -> current_transformation/3(w)
  [iu_inverter] -> sample_hold_normalization/1(iu)  "iu"
  sample_hold_normalization/1(iu_pu) -> current_transformation/1(u)
  [iv_inverter] -> sample_hold_normalization/2(iv)  "iv"
  [iw_inverter] -> sample_hold_normalization/3(iw)  "iw"
  phase/1 -> current_transformation/4(phase)
  sample_hold_normalization/2(iv_pu) -> current_transformation/2(v)

== system ps_model/control_system/phase_gen ==
  Constant4 : Constant  Value=2*pi*fnom
  Sum4 : Sum  SaturateOnIntegerOverflow=on
  Unit Delay1 : UnitDelay  SampleTime=ts_inv  HasFrameUpgradeWarning=on
  bounder1 : MATLAB Function  TreatAsAtomicUnit=on  SystemSampleTime=ts_inv
  kp2 : Gain  Gain=ts_inv  SaturateOnIntegerOverflow=on  OutDataTypeStr=Inherit: Same as input  ParamDataTypeStr=Inherit: Same as input
  electrical_phase : Outport
  wires:
  Unit Delay1/1 -> Sum4/2
  Constant4/1 -> kp2/1
  kp2/1 -> Sum4/1
  bounder1/1(y) -> Unit Delay1/1, electrical_phase/1
  Sum4/1 -> bounder1/1(u)

== system ps_model/control_system/scalar_voltage_control ==
  1/Ti1 : Gain  Gain=-1  SaturateOnIntegerOverflow=on  OutDataTypeStr=Inherit: Same as input  ParamDataTypeStr=Inherit: Same as input
  1/Ti2 : Gain  Gain=-1  SaturateOnIntegerOverflow=on  OutDataTypeStr=Inherit: Same as input  ParamDataTypeStr=Inherit: Same as input
  Constant : Constant  Value=1.5
  Constant1 : Constant
  Constant2 : Constant  Value=0  SampleTime=ts_inv
  Math Function{,1..3} (4 alike) : Math  Operator=magnitude^2  SignedPower=on
  Min : MinMax  Inputs=2
  Sqrt : Sqrt
  Sqrt1 : Sqrt
  Sum1 : Sum  Inputs=|++
  Sum9 : Sum  Inputs=|++
  ctrl_out_i/ctrl_out_u : Scope  NumInputPorts=2
  i/i_ref : Scope  NumInputPorts=2
  pi_ctrl_i : Subsystem  mask{kp=kp_i, ki=ki_i, ts=ts_inv, sat_pos=1, sat_neg=0}
  pi_ctrl_u : Subsystem  mask{kp=kp_u, ki=ki_u, ts=ts_inv, sat_pos=1, sat_neg=0}
  u/u_ref : Scope  NumInputPorts=2
  u_ctrl_outs : Scope  NumInputPorts=2
  d : Outport
  q : Outport  Port=2
  wires:
  [u_alpha_out_pu] -> Math Function1/1
  Math Function/1 -> Sum9/1
  Sum9/1 -> Sqrt/1
  [u_beta_out_pu] -> Math Function/1
  Math Function1/1 -> Sum9/2
  Min/1 -> 1/Ti2/1
  1/Ti1/1 -> q/1, u_ctrl_outs/2
  Constant1/1 -> u/u_ref/1, pi_ctrl_u/2(xref)
  Sqrt/1 -> u/u_ref/2, pi_ctrl_u/1(x)
  Sqrt1/1 -> pi_ctrl_i/1(x), i/i_ref/2
  Constant/1 -> i/i_ref/1, pi_ctrl_i/2(xref)
  Math Function3/1 -> Sum1/2
  [i_beta_inverter_pu] -> Math Function2/1
  Sum1/1 -> Sqrt1/1
  Math Function2/1 -> Sum1/1
  [i_alpha_inverter_pu] -> Math Function3/1
  Constant2/1 -> 1/Ti1/1
  pi_ctrl_u/1(u) -> Min/2, ctrl_out_i/ctrl_out_u/2  "ctrl_out_u"
  pi_ctrl_i/1(u) -> ctrl_out_i/ctrl_out_u/1, Min/1  "ctrl_out_i"
  1/Ti2/1 -> u_ctrl_outs/1, d/1

== system ps_model/control_system/voltage_measure ==
  phase : Inport
  Demux : Demux  Outputs=3
  sample_hold_normalization : Subsystem
  voltage_transformation : Subsystem
  wires:
  sample_hold_normalization/2(uv_pu) -> voltage_transformation/2(v)
  phase/1 -> voltage_transformation/4(phase)
  Demux/3 -> sample_hold_normalization/3(iw)  "uout_w"
  Demux/2 -> sample_hold_normalization/2(iv)  "uout_v"
  sample_hold_normalization/1(uu_pu) -> voltage_transformation/1(u)
  Demux/1 -> sample_hold_normalization/1(iu)  "uout_u"
  sample_hold_normalization/3(uw_pu) -> voltage_transformation/3(w)
  [uout2_uvw] -> Demux/1  "uout_uvw"

== system ps_model/grid/grid_emulator ==
  Controlled Voltage Source : fl_lib/Electrical/Electrical Sources/Controlled Voltage Source
  Controlled Voltage Source1 : fl_lib/Electrical/Electrical Sources/Controlled Voltage Source
  Controlled Voltage Source2 : fl_lib/Electrical/Electrical Sources/Controlled Voltage Source
  Electrical Reference : fl_lib/Electrical/Electrical Elements/Electrical Reference
  Inductor : fl_lib/Electrical/Electrical Elements/Inductor  l=10e-6 H  r=0 Ohm  g=1e-3 1/Ohm  i_specify=off  i_priority=None  i=0 A  i_nominal_specify=off  i_nominal_unit=A  i_nominal_value=1  v_specify=off  v_priority=None  v=0 V  v_nominal_specify=off  v_nominal_unit=V  v_nominal_value=1  i_L_specify=off  i_L_priority=High  i_L=0 A  i_L_nominal_specify=off  i_L_nominal_unit=A  i_L_nominal_value=1
  Inductor1 : fl_lib/Electrical/Electrical Elements/Inductor  l=10e-6 H  r=0 Ohm  g=1e-3 1/Ohm  i_specify=off  i_priority=None  i=0 A  i_nominal_specify=off  i_nominal_unit=A  i_nominal_value=1  v_specify=off  v_priority=None  v=0 V  v_nominal_specify=off  v_nominal_unit=V  v_nominal_value=1  i_L_specify=off  i_L_priority=High  i_L=0 A  i_L_nominal_specify=off  i_L_nominal_unit=A  i_L_nominal_value=1
  Inductor2 : fl_lib/Electrical/Electrical Elements/Inductor  l=10e-6 H  r=0 Ohm  g=1e-3 1/Ohm  i_specify=off  i_priority=None  i=0 A  i_nominal_specify=off  i_nominal_unit=A  i_nominal_value=1  v_specify=off  v_priority=None  v=0 V  v_nominal_specify=off  v_nominal_unit=V  v_nominal_value=1  i_L_specify=off  i_L_priority=High  i_L=0 A  i_L_nominal_specify=off  i_L_nominal_unit=A  i_L_nominal_value=1
  Inductor3 : fl_lib/Electrical/Electrical Elements/Inductor  l=1e-6 H  r=0 Ohm  g=1e-3 1/Ohm  i_specify=off  i_priority=None  i=0 A  i_nominal_specify=off  i_nominal_unit=A  i_nominal_value=1  v_specify=off  v_priority=None  v=0 V  v_nominal_specify=off  v_nominal_unit=V  v_nominal_value=1  i_L_specify=off  i_L_priority=High  i_L=0 A  i_L_nominal_specify=off  i_L_nominal_unit=A  i_L_nominal_value=1
  Inductor4 : fl_lib/Electrical/Electrical Elements/Inductor  l=1e-6 H  r=0 Ohm  g=1e-3 1/Ohm  i_specify=off  i_priority=None  i=0 A  i_nominal_specify=off  i_nominal_unit=A  i_nominal_value=1  v_specify=off  v_priority=None  v=0 V  v_nominal_specify=off  v_nominal_unit=V  v_nominal_value=1  i_L_specify=off  i_L_priority=High  i_L=0 A  i_L_nominal_specify=off  i_L_nominal_unit=A  i_L_nominal_value=1
  Inductor5 : fl_lib/Electrical/Electrical Elements/Inductor  l=1e-6 H  r=0 Ohm  g=1e-3 1/Ohm  i_specify=off  i_priority=None  i=0 A  i_nominal_specify=off  i_nominal_unit=A  i_nominal_value=1  v_specify=off  v_priority=None  v=0 V  v_nominal_specify=off  v_nominal_unit=V  v_nominal_value=1  i_L_specify=off  i_L_priority=High  i_L=0 A  i_L_nominal_specify=off  i_L_nominal_unit=A  i_L_nominal_value=1
  Simulink-PS Converter : nesl_utility/Simulink-PS Converter  PhysicalDomain=network_engine_domain  SubClassName=ps_input  LeftPortType=input  RightPortType=output  PseudoPeriodic=off  Frequencies=[]  NoiseDistribution=none  NoiseParameters=[]  Unit=V  AffineConversion=off  FilteringAndDerivatives=provide  SimscapeFilterOrder=1  InputFilterTimeConstant=0.001  UdotUserProvided=0
  Simulink-PS Converter1 : nesl_utility/Simulink-PS Converter  PhysicalDomain=network_engine_domain  SubClassName=ps_input  LeftPortType=input  RightPortType=output  PseudoPeriodic=off  Frequencies=[]  NoiseDistribution=none  NoiseParameters=[]  Unit=V  AffineConversion=off  FilteringAndDerivatives=provide  SimscapeFilterOrder=1  InputFilterTimeConstant=0.001  UdotUserProvided=0
  Simulink-PS Converter2 : nesl_utility/Simulink-PS Converter  PhysicalDomain=network_engine_domain  SubClassName=ps_input  LeftPortType=input  RightPortType=output  PseudoPeriodic=off  Frequencies=[]  NoiseDistribution=none  NoiseParameters=[]  Unit=V  AffineConversion=off  FilteringAndDerivatives=provide  SimscapeFilterOrder=1  InputFilterTimeConstant=0.001  UdotUserProvided=0
  Solver Configuration : nesl_utility/Solver Configuration  PhysicalDomain=network_engine_domain  SubClassName=solver  LeftPortType=input  RightPortType=generic  Tones=[]  Harmonics=[]  SimulateNoise=off  Profile=off  UseLocalSampling=off  EnableSwitchedLinearOptims=on  FrequencyDomain=off  UseCCode=off  RelTol=0.001  AbsTol=0.001  MinStep=1e-09  ToWorkspace=off  RevertToSquareIcSolve=off  NumHomotopyIterations=100  PhasorMode=off  PhasorModeNumHarmonics=1  ConsistencySolver=NEWTON_XTOL_AFTER_FTOL  IndexReductionMethod=DerivativeReplacement  DoDC=on  ResidualTolerance=1e-09  ConsistencyTolSource=GLOBAL  ConsistencyAbsTol=0.001  ConsistencyRelTol=0.001  ConsistencyTolFactor=0.001  UseLocalSolver=on  LocalSolverChoice=NE_BACKWARD_EULER_ADVANCER  ResolveIndetEquations=on  FunctionEvalNumThread=1  LocalSolverSampleTime=tc  DoFixedCost=on  MaxNonlinIter=3  MaxModeIter=2  ComputeImpulses=off  ImpulseIterations=2  LinearAlgebra=auto  LinearAlgebraNumThread=0  EquationFormulation=NE_TIME_EF  DelaysMemoryBudget=1024  AutomaticFiltering=on  FilteringTimeConstant=0.001  PartitionStorageMethod=AS_NEEDED  PartitionMemoryBudget=1024  PartitionMethod=ROBUST  MultibodyUseLocalSolver=off  MultibodyLocalSolverChoice=ODE1  MultibodyLocalSolverSampleTime=0.001
  grid_emulator : Subsystem
  threephase_vi_measures_mv : Subsystem
  u1 : PMIOPort  Side=Right
  u2 : PMIOPort  Port=2  Side=Right
  u3 : PMIOPort  Port=3  Side=Right
  wires:
  grid_emulator/2(Vmb) -> Simulink-PS Converter1/1
  grid_emulator/3(Vmc) -> Simulink-PS Converter2/1
  grid_emulator/1(Vma) -> Simulink-PS Converter/1
  connections:
  Simulink-PS Converter/RConn1 -- Controlled Voltage Source/RConn1
  Simulink-PS Converter1/RConn1 -- Controlled Voltage Source1/RConn1
  Simulink-PS Converter2/RConn1 -- Controlled Voltage Source2/RConn1
  Electrical Reference/LConn1 -- Solver Configuration/RConn1 -- Controlled Voltage Source/RConn2 -- Controlled Voltage Source1/RConn2 -- Controlled Voltage Source2/RConn2
  Controlled Voltage Source/LConn1 -- Inductor/LConn1
  Inductor1/LConn1 -- Controlled Voltage Source1/LConn1
  Inductor2/LConn1 -- Controlled Voltage Source2/LConn1
  u1/RConn1 -- Inductor3/RConn1
  u2/RConn1 -- Inductor4/RConn1
  u3/RConn1 -- Inductor5/RConn1
  Inductor/RConn1 -- threephase_vi_measures_mv/LConn1
  Inductor1/RConn1 -- threephase_vi_measures_mv/LConn2
  Inductor2/RConn1 -- threephase_vi_measures_mv/LConn3
  Inductor3/LConn1 -- threephase_vi_measures_mv/RConn1
  Inductor4/LConn1 -- threephase_vi_measures_mv/RConn2
  Inductor5/LConn1 -- threephase_vi_measures_mv/RConn3

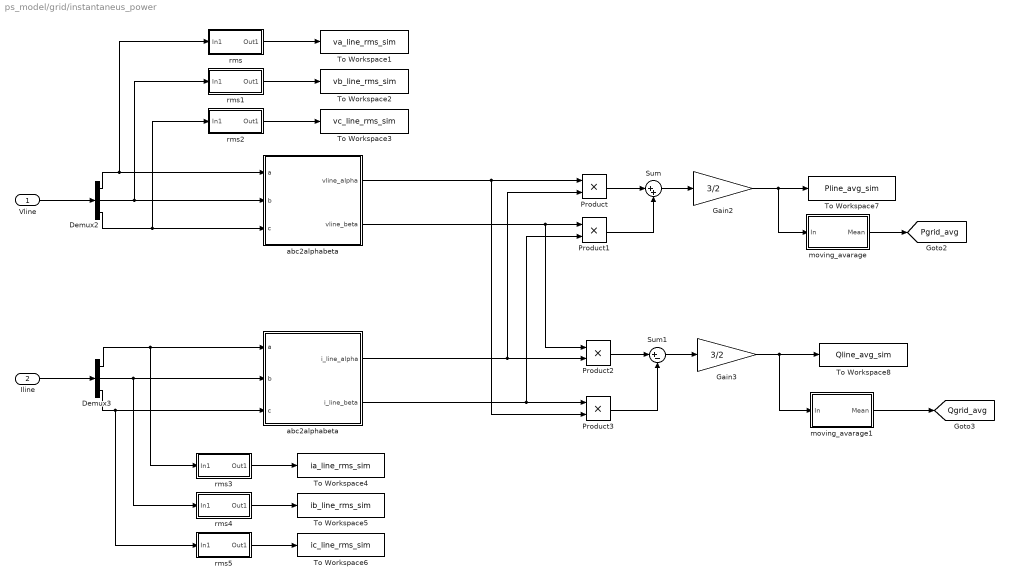
== system ps_model/grid/instantaneus_power ==
  Vline : Inport
  Iline : Inport  Port=2
  Demux2 : Demux  Outputs=3
  Demux3 : Demux  Outputs=3
  Gain2 : Gain  Gain=3/2
  Gain3 : Gain  Gain=3/2
  Product{,1..3} (4 alike) : Product  RndMeth=Zero
  Sum : Sum  Inputs=|++
  Sum1 : Sum  Inputs=|+-
  To Workspace1 : ToWorkspace  VariableName=va_line_rms_sim  SampleTime=ts_afe
      settings: MaxDataPoints=Ns_afe
  To Workspace2 : ToWorkspace  VariableName=vb_line_rms_sim  SampleTime=ts_afe
      settings: MaxDataPoints=Ns_afe
  To Workspace3 : ToWorkspace  VariableName=vc_line_rms_sim  SampleTime=ts_afe
      settings: MaxDataPoints=Ns_afe
  To Workspace4 : ToWorkspace  VariableName=ia_line_rms_sim  SampleTime=ts_afe
      settings: MaxDataPoints=Ns_afe
  To Workspace5 : ToWorkspace  VariableName=ib_line_rms_sim  SampleTime=ts_afe
      settings: MaxDataPoints=Ns_afe
  To Workspace6 : ToWorkspace  VariableName=ic_line_rms_sim  SampleTime=ts_afe
      settings: MaxDataPoints=Ns_afe
  To Workspace7 : ToWorkspace  VariableName=Pline_avg_sim  SampleTime=ts_afe
      settings: MaxDataPoints=Ns_afe
  To Workspace8 : ToWorkspace  VariableName=Qline_avg_sim  SampleTime=ts_afe
      settings: MaxDataPoints=Ns_afe
  abc2alphabeta : Subsystem
  "abc2alphabeta " : Subsystem
  moving_avarage : Subsystem
  moving_avarage1 : Subsystem
  rms : Subsystem
  rms1 : Subsystem
  rms2 : Subsystem
  rms3 : Subsystem
  rms4 : Subsystem
  rms5 : Subsystem
  tag scope: Pgrid_avg=global, Qgrid_avg=global
  wires:
  Gain3/1 -> moving_avarage1/1(In), To Workspace8/1
  Gain2/1 -> moving_avarage/1(In), To Workspace7/1
  Demux2/1 -> rms/1(In1), abc2alphabeta/1(a)
  Vline/1 -> Demux2/1
  Iline/1 -> Demux3/1
  abc2alphabeta/2(vline_beta) -> Product1/1, Product2/1
  "abc2alphabeta "/2(i_line_beta) -> Product3/1, Product1/2
  abc2alphabeta/1(vline_alpha) -> Product/1, Product3/2
  "abc2alphabeta "/1(i_line_alpha) -> Product2/2, Product/2
  Product/1 -> Sum/1
  Product1/1 -> Sum/2
  Product2/1 -> Sum1/1
  Product3/1 -> Sum1/2
  Sum1/1 -> Gain3/1
  Sum/1 -> Gain2/1
  Demux2/2 -> rms1/1(In1), abc2alphabeta/2(b)
  Demux2/3 -> rms2/1(In1), abc2alphabeta/3(c)
  Demux3/1 -> "abc2alphabeta "/1(a), rms3/1(In1)
  Demux3/2 -> "abc2alphabeta "/2(b), rms4/1(In1)
  Demux3/3 -> rms5/1(In1), "abc2alphabeta "/3(c)
  moving_avarage/1(Mean) -> [Pgrid_avg]
  moving_avarage1/1(Mean) -> [Qgrid_avg]
  rms/1(Out1) -> To Workspace1/1
  rms2/1(Out1) -> To Workspace3/1
  rms1/1(Out1) -> To Workspace2/1
  rms5/1(Out1) -> To Workspace6/1
  rms4/1(Out1) -> To Workspace5/1
  rms3/1(Out1) -> To Workspace4/1

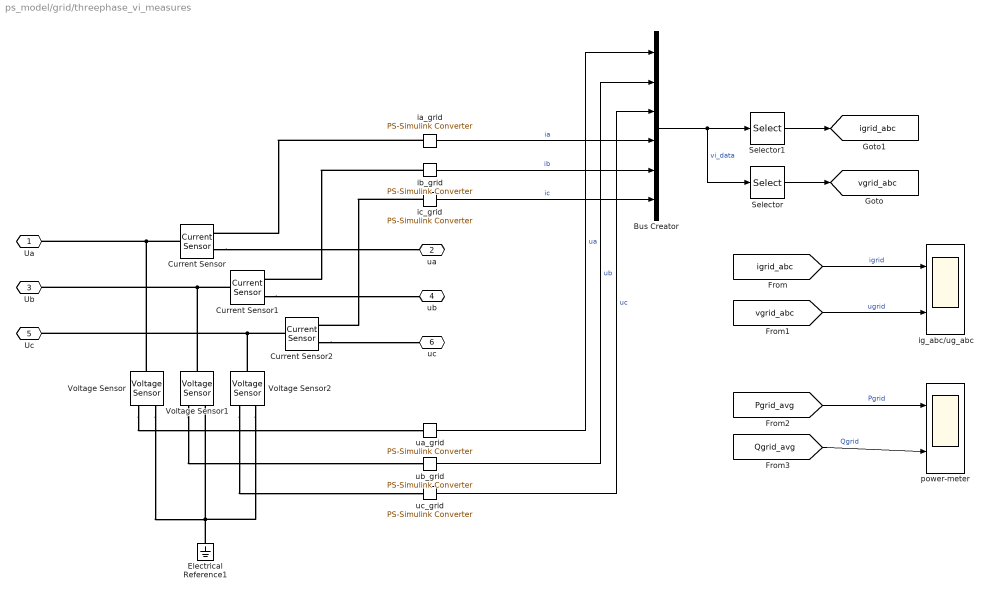
== system ps_model/grid/threephase_vi_measures ==
  Bus Creator : BusCreator  Inputs=6
  Current Sensor : fl_lib/Electrical/Electrical Sensors/Current Sensor
  Current Sensor1 : fl_lib/Electrical/Electrical Sensors/Current Sensor
  Current Sensor2 : fl_lib/Electrical/Electrical Sensors/Current Sensor
  Electrical Reference1 : fl_lib/Electrical/Electrical Elements/Electrical Reference
  Selector : Selector  InputPortWidth=6  IndexOptions=Index vector (dialog)  Indices=[1 2 3]  OutputSizes=1
  Selector1 : Selector  InputPortWidth=6  IndexOptions=Index vector (dialog)  Indices=[4 5 6]  OutputSizes=1
  Voltage Sensor : fl_lib/Electrical/Electrical Sensors/Voltage Sensor
  Voltage Sensor1 : fl_lib/Electrical/Electrical Sensors/Voltage Sensor
  Voltage Sensor2 : fl_lib/Electrical/Electrical Sensors/Voltage Sensor
  ia_grid : nesl_utility/PS-Simulink Converter  PhysicalDomain=network_engine_domain  SubClassName=ps_output  LeftPortType=input  RightPortType=output  PseudoPeriodic=off  Frequencies=[]  VectorFormat=1-D array  Unit=A  AffineConversion=off
  ib_grid : nesl_utility/PS-Simulink Converter  PhysicalDomain=network_engine_domain  SubClassName=ps_output  LeftPortType=input  RightPortType=output  PseudoPeriodic=off  Frequencies=[]  VectorFormat=1-D array  Unit=A  AffineConversion=off
  ic_grid : nesl_utility/PS-Simulink Converter  PhysicalDomain=network_engine_domain  SubClassName=ps_output  LeftPortType=input  RightPortType=output  PseudoPeriodic=off  Frequencies=[]  VectorFormat=1-D array  Unit=A  AffineConversion=off
  ig_abc/ug_abc : Scope  NumInputPorts=2
  power-meter : Scope  NumInputPorts=2
  ua_grid : nesl_utility/PS-Simulink Converter  PhysicalDomain=network_engine_domain  SubClassName=ps_output  LeftPortType=input  RightPortType=output  PseudoPeriodic=off  Frequencies=[]  VectorFormat=1-D array  Unit=V  AffineConversion=off
  ub_grid : nesl_utility/PS-Simulink Converter  PhysicalDomain=network_engine_domain  SubClassName=ps_output  LeftPortType=input  RightPortType=output  PseudoPeriodic=off  Frequencies=[]  VectorFormat=1-D array  Unit=V  AffineConversion=off
  uc_grid : nesl_utility/PS-Simulink Converter  PhysicalDomain=network_engine_domain  SubClassName=ps_output  LeftPortType=input  RightPortType=output  PseudoPeriodic=off  Frequencies=[]  VectorFormat=1-D array  Unit=V  AffineConversion=off
  Ua : PMIOPort  Side=Left
  ua : PMIOPort  Port=2  Side=Right
  Ub : PMIOPort  Port=3  Side=Left
  ub : PMIOPort  Port=4  Side=Right
  Uc : PMIOPort  Port=5  Side=Left
  uc : PMIOPort  Port=6  Side=Right
  tag scope: igrid_abc=global, vgrid_abc=global
  wires:
  Bus Creator/1 -> Selector1/1, Selector/1  "vi_data"
  Selector/1 -> [vgrid_abc]
  ib_grid/1 -> Bus Creator/5  "ib"
  ia_grid/1 -> Bus Creator/4  "ia"
  ic_grid/1 -> Bus Creator/6  "ic"
  ua_grid/1 -> Bus Creator/1  "ua"
  ub_grid/1 -> Bus Creator/2  "ub"
  uc_grid/1 -> Bus Creator/3  "uc"
  Selector1/1 -> [igrid_abc]
  [vgrid_abc] -> ig_abc/ug_abc/2  "ugrid"
  [igrid_abc] -> ig_abc/ug_abc/1  "igrid"
  [Pgrid_avg] -> power-meter/1  "Pgrid"
  [Qgrid_avg] -> power-meter/2  "Qgrid"
  connections:
  Current Sensor1/LConn1 -- Ub/RConn1 -- Voltage Sensor1/LConn1
  Electrical Reference1/LConn1 -- Voltage Sensor/RConn2 -- Voltage Sensor2/RConn2 -- Voltage Sensor1/RConn2
  Voltage Sensor/RConn1 -- ua_grid/LConn1
  Current Sensor/RConn2 -- ua/RConn1
  Voltage Sensor1/RConn1 -- ub_grid/LConn1
  Voltage Sensor2/LConn1 -- Current Sensor2/LConn1 -- Uc/RConn1
  Current Sensor/LConn1 -- Ua/RConn1 -- Voltage Sensor/LConn1
  Current Sensor1/RConn2 -- ub/RConn1
  Voltage Sensor2/RConn1 -- uc_grid/LConn1
  ib_grid/LConn1 -- Current Sensor1/RConn1
  ia_grid/LConn1 -- Current Sensor/RConn1
  ic_grid/LConn1 -- Current Sensor2/RConn1
  Current Sensor2/RConn2 -- uc/RConn1
